simulink library "vel_controller_lib"  (R2018b)
settings: Solver=VariableStepAuto  StartTime=0.0  StopTime=10.0  RelTol=1e-3
undefined symbols (not defined in the file): thrust_feedforward, vel_param_xy, vel_param_z, vel_sample_h, vel_sat_angle
libraries: $bdroot x1
settings Model: Creator=sebbe  LastModifiedBy=Pontus

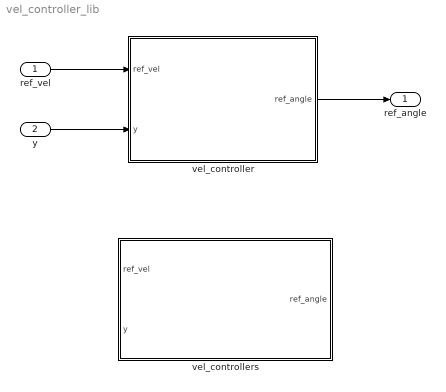
== system vel_controller_lib ==
  ref_vel : Inport  PortDimensions=[3]
  y : Inport  Port=2
  vel_controller : Subsystem
  vel_controllers : Subsystem  TreatAsAtomicUnit=on
  ref_angle : Outport
  wires:
  ref_vel/1 -> vel_controller/1(ref_vel)
  y/1 -> vel_controller/2(y)
  vel_controller/1(ref_angle) -> ref_angle/1

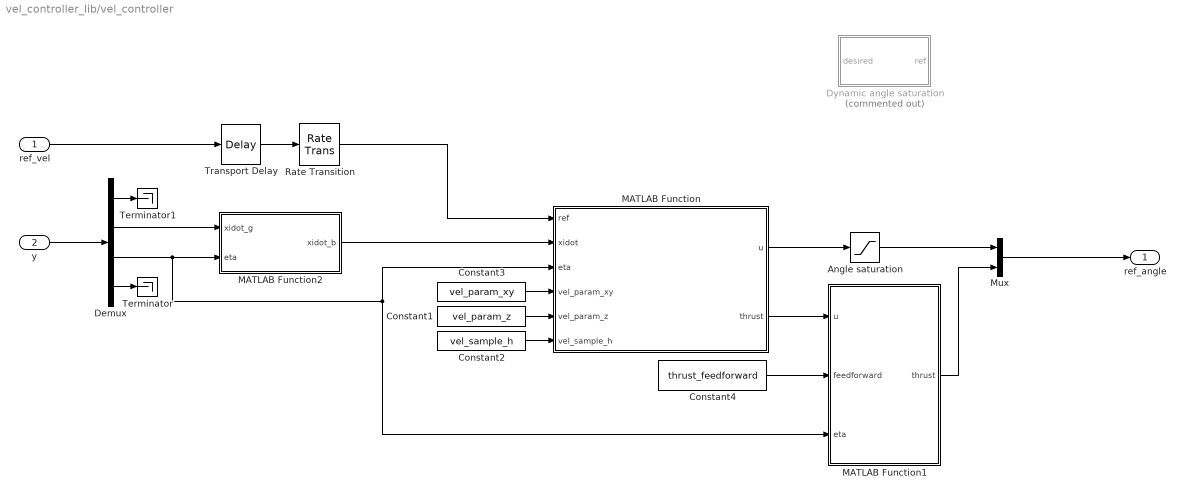
== system vel_controller_lib/vel_controller ==
  ref_vel : Inport
  y : Inport  Port=2
  Angle saturation : Saturate  UpperLimit=vel_sat_angle  LowerLimit=-vel_sat_angle
  Constant1 : Constant  Value=vel_param_z
  Constant2 : Constant  Value=vel_sample_h
  Constant3 : Constant  Value=vel_param_xy
  Constant4 : Constant  Value=thrust_feedforward
  Demux : Demux
  Dynamic angle saturation : MATLAB Function  Commented=on  TreatAsAtomicUnit=on
  MATLAB Function : MATLAB Function  TreatAsAtomicUnit=on  SystemSampleTime=vel_sample_h
  MATLAB Function1 : MATLAB Function  TreatAsAtomicUnit=on
  MATLAB Function2 : MATLAB Function  TreatAsAtomicUnit=on
  Mux : Mux  Inputs=[3 1]
  Rate Transition : RateTransition  InitialCondition=[0; 0; 0]  OutPortSampleTime=0.01
  Terminator : Terminator
  Terminator1 : Terminator
  Transport Delay : TransportDelay  DelayTime=0.005  InitialOutput=[0; 0; 0]
  ref_angle : Outport
  wires:
  Angle saturation/1 -> Mux/1
  Rate Transition/1 -> MATLAB Function/1(ref)
  ref_vel/1 -> Transport Delay/1
  Transport Delay/1 -> Rate Transition/1
  MATLAB Function1/1(thrust) -> Mux/2
  MATLAB Function/2(thrust) -> MATLAB Function1/1(u)
  MATLAB Function/1(u) -> Angle saturation/1
  Constant4/1 -> MATLAB Function1/2(feedforward)
  Constant2/1 -> MATLAB Function/6(vel_sample_h)
  Demux/4 -> Terminator/1
  Constant3/1 -> MATLAB Function/4(vel_param_xy)
  Demux/2 -> MATLAB Function2/1(xidot_g)
  Mux/1 -> ref_angle/1
  Constant1/1 -> MATLAB Function/5(vel_param_z)
  Demux/3 -> MATLAB Function1/3(eta), MATLAB Function/3(eta), MATLAB Function2/2(eta)
  MATLAB Function2/1(xidot_b) -> MATLAB Function/2(xidot)
  Demux/1 -> Terminator1/1
  y/1 -> Demux/1

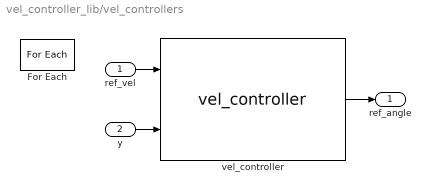
== system vel_controller_lib/vel_controllers ==
  ref_vel : Inport  Partition=on  PartitionDimension=2  PartitionWidth=1  PartitionOffset=0
  y : Inport  Port=2  Partition=on  PartitionDimension=2  PartitionWidth=1  PartitionOffset=0
  For Each : ForEach  DisableCoverage=on  IndexMode=One-based
  vel_controller : $bdroot/vel_controller  SystemSampleTime=-1
  ref_angle : Outport  ConcatenationDimension=2
  wires:
  ref_vel/1 -> vel_controller/1
  y/1 -> vel_controller/2
  vel_controller/1 -> ref_angle/1

== matlab function vel_controller_lib/vel_controller/MATLAB Function ==
  data: ref input; u output size=[3]; xidot input; eta input; vel_param_xy input; vel_param_z input; vel_sample_h input; thrust output size=1
function [u, thrust]= velocitycontrolPID(ref, xidot, eta, vel_param_xy, vel_param_z, vel_sample_h)
    persistent integ prev_error
    if isempty(integ)
        integ = [0;0;0];
    end
    if isempty(prev_error)
        prev_error = [0;0;0];
    end
    
    % Remap desired velocity from inertial to body frame
    R = eta2Rgb(eta, 0);
    ref = R*ref;
    error = ref - xidot;
    
    % Shift roll and pitch as X_error = pitch & Y_error = -roll
    error = [-error(2); error(1); error(3)];
    
    % Retrieve parameters
    KP = [vel_param_xy(1); vel_param_xy(1); vel_param_z(1)];
    KI = [vel_param_xy(2); vel_param_xy(2); vel_param_z(2)];
    KD = [vel_param_xy(3); vel_param_xy(3); vel_param_z(3)];
    i_sat = vel_param_z(4);
    
    out = [0;0;0];
    
    out = out + KP.*error;
    
    integ = integ + error*vel_sample_h;
    integ = max(-i_sat, min(i_sat, integ)); % Limit to i_sat
    out = out + integ.*KI;
    
    deriv = (error-prev_error)/vel_sample_h;
    out = out + deriv.*KD;
    prev_error = error;
    
    u = [out(1); out(2); 0];
    thrust = out(3);
end

== matlab function vel_controller_lib/vel_controller/Dynamic angle saturation ==
  data: desired input size=[3]; ref output size=[3]; vel_sat_angle parameter size=1
function ref = fcn(desired, vel_sat_angle)
% ref = saturate_angle(desired, vel_sat_angle);
%ref = desired;
end

== matlab function vel_controller_lib/vel_controller/MATLAB Function1 ==
  data: u input; thrust output; feedforward input; eta input
function thrust = thrust_feedforward(u, feedforward, eta)

%thrust = (feedforward + 5000*u)/(cos(eta(1))*cos(eta(2)));
%thrust = (feedforward + 1000*u)/(cos(eta(1))*cos(eta(2)));
thrust = (feedforward + 1000*u);

end

== matlab function vel_controller_lib/vel_controller/MATLAB Function2 ==
  data: xidot_g input size=[3]; xidot_b output size=[3]; eta input size=[3]
function xidot_b = xidot_global2body(xidot_g, eta)
    R = eta2Rgb(eta, 0);
    xidot_b = R*xidot_g;
end
